simulink model "chydr_s_Wch"  (Simulink 8.9)
settings: Solver=ode45  StartTime=0.0  StopTime=10  MaxStep=10  MinStep=0.0001  RelTol=1e-6  AbsTol=1e-6  EnableMultiTasking=on
values from neighbouring files (symbols this model uses):
  kw = 0.5    [datahydr_pprTf5.mat]    (also in initchydr_yuwch.m)
  Ta = 10    [datahydr_pprTf5.mat]    (also in initchydr_yuwch.m)
  TI = 0.3    [datahydr_pprTf5.mat]    (also in initchydr_yuwch.m)
  Tw = 1    [datahydr_pprTf5.mat]    (also in initchydr_yuwch.m)
settings Model: SuppressorTable=22 serialization::archive 11 0 6 0 0 0 11 0  Creator=pchevrel  LastModifiedBy=pl
settings DataIOCC: SaveOutput=off  SaveTime=off  SignalLoggingName=sigsOut
settings OptimizationCC: ExpressionDepthLimit=2147483647  InitFltsAndDblsToZero=on
settings DebuggingCC: SaveWithParameterizedLinksMsg=none  SignalResolutionControl=TryResolveAllWithWarning  MultiTaskDSMMsg=warning  MultiTaskCondExecSysMsg=none  StrictBusMsg=None
settings HardwareCC: TargetUnknown=on
settings GRTTargetCC: TargetFcnLib=ansi_tfl_tmw.mat  GeneratePreprocessorConditionals=Use local settings

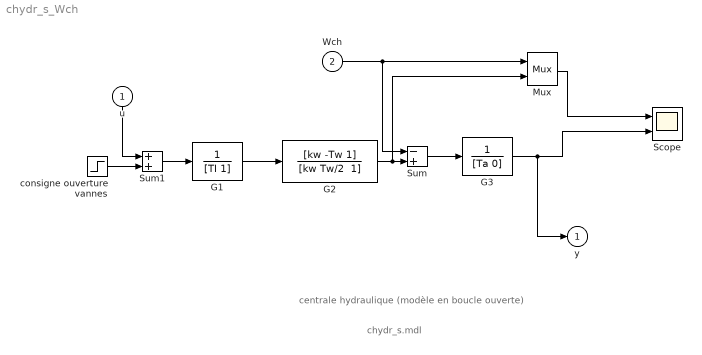
== system chydr_s_Wch ==
  note: chydr_s.mdl
  note: centrale hydraulique (modèle en boucle ouverte)
  u : Inport
  Wch : Inport  Port=2
  G1 : TransferFcn  Denominator=[TI 1]
  G2 : TransferFcn  Numerator=[kw -Tw 1]  Denominator="[kw Tw/2  1]"
  G3 : TransferFcn  Denominator=[Ta 0]
  Mux : Mux  Inputs=2
  Scope : Scope  NumInputPorts=2
  Sum : Sum  Inputs=-+  SaturateOnIntegerOverflow=on  InputSameDT=on  OutDataTypeStr=Inherit: Same as first input
  Sum1 : Sum  SaturateOnIntegerOverflow=on  InputSameDT=on  OutDataTypeStr=Inherit: Same as first input
  consigne ouverture vannes : Step  Time=0  After=100  SampleTime=0
  y : Outport
  wires:
  G2/1 -> Sum/2, Mux/2
  Sum/1 -> G3/1
  G3/1 -> y/1, Scope/2
  G1/1 -> G2/1
  Wch/1 -> Sum/1, Mux/1
  Mux/1 -> Scope/1
  Sum1/1 -> G1/1
  consigne ouverture vannes/1 -> Sum1/2
  u/1 -> Sum1/1
